simulink model "RoboBoat_SLAM_6_29"  (R2014a)
settings: Solver=FixedStepDiscrete  StartTime=0.0  StopTime=inf  FixedStep=.1  RelTol=1e-3
undefined symbols (not defined in the file): Com1, Com2, Com3, Com4, DiscIntNeverNeededParam, standard
libraries: xpcseriallib x29, visiontextngfix x25, simulink x21, slrtlib x7, speedgoatlib_IO102 x5, speedgoatlib x1
(part 5 of 6)

== matlab function RoboBoat_SLAM_6_29/Main FSM/Obstacle Navigation1/Task Option1/Message Composer ==
  data: taskStrInit input; taskStrAdj output
function taskStrAdj = composeMessage(taskStrInit)
%Written by Anderson Lebbad on August 9, 2013
%Last Edited: Edward Zhu on June 2, 2014

%This function adjusts the length of a vector to a set value by filling
%the remaining space with 0's. This is necessary for data store objects
%that have a fixed size for the memory allocation, but a variable length
%input.

%Length of message packet
strLength = 8;

%Size of text in message
taskStrLength = size(taskStrInit,1);

%Pad end of text with zeros
taskStrAdj = [taskStrInit' zeros(1,strLength-taskStrLength)];

== matlab function RoboBoat_SLAM_6_29/Main FSM/Obstacle Navigation1/GPS: Center/Orient/Within Range ==
  data: DesiredHeading input; Finished output; Compass input
function Finished = OrientLocked(DesiredHeading, Compass)

%Written by Anderson Lebbad on July 22, 2013
%Last Edited:

%This function checks to see if the target heading has been reached and 
%sends a finished signal when it has.

HeadingDiff = DesiredHeading - Compass;

%Sets the range for the difference angle to be -180 to +180
if HeadingDiff > 180
    HeadingDiff = HeadingDiff - 360;
elseif HeadingDiff < -180
    HeadingDiff = HeadingDiff + 360;
end

%If the Heading is within 3 degrees, the angle is close enough to send a
%finished signal
if abs(HeadingDiff) < 3
    Finished = 1;
else
    Finished = 0;
end

== matlab function RoboBoat_SLAM_6_29/Main FSM/Obstacle Navigation1/Obstacle Navigation/Dodge/Nav Logic ==
  data: CurrentHeading input; Dist input; Ang input; ObstDist output; RPM output; DesiredHeading output; Timer input; Timeout input; DodgeIncomplete output
 function [ObstDist, RPM, DesiredHeading, DodgeIncomplete] = NavLogic(CurrentHeading,...
    Dist, Ang, Timer, Timeout)

%Written by Anderson Lebbad on August 20, 2013
%Last Edited by:

%Determines the signals for driving through the buoy channel based on the
%bounding box and centroid signals from both the red and green detection
%blocks.

persistent TimeLastFound heldHeading

ObstDist = Dist / 100;

if isempty(TimeLastFound) && isempty(heldHeading)
    TimeLastFound = 0;
    heldHeading = CurrentHeading;
end

if ObstDist > 0 && ObstDist <= 2
    %Buffer for single buoy offset is the angle to twice the boat's width off of the
    %center of the buoy
    BoatWidth = .75;
    Buffer = atan(2 * BoatWidth / ObstDist) * 180 / pi;
    
    if Ang < 0
        ObstOffset = Ang + Buffer;
    else
        ObstOffset = Ang - Buffer;
    end
    
    DesiredHeading = mod(CurrentHeading + ObstOffset, 360);
    RPM = 2800;
    
    TimeLastFound = Timer;
    heldHeading = CurrentHeading;
    
    DodgeIncomplete = 1;
    
else
    DesiredHeading = heldHeading;
    RPM = 2800;
    
    if Timer-TimeLastFound < Timeout
        DodgeIncomplete = 1;
    else
        DodgeIncomplete = 0;
    end

end

== matlab function RoboBoat_SLAM_6_29/Sensors/1020 Comms/Data Update2 ==
  data: Valid input; ControlMode input; V output; C output; L output; A output; Data input; D1 output; D2 output; D3 output; D4 output; D5 output; D6 output; D7 output; D8 output; D9 output; D10 output; D11 output; D12 output; D13 output; D14 output; D15 output; D16 output; D17 output; D18 output; D19 output; D20 output; D21 output; D22 output; D23 output; D24 output; Activate input
function [V,C,L,A,D1,D2,D3,D4,D5,D6,D7,D8,D9,D10,D11,D12,D13,D14,D15,D16,D17,...
    D18,D19,D20,D21,D22,D23,D24] = dataSplit(Valid,ControlMode,Data,Activate)
%Written by Anderson Lebbad on August 10, 2014
%Last Edited by: Anderson Lebbad on September 11, 2014

%This function splits the data vector into the twelve channels it is
%composed of for communication

persistent HoldData

if isempty(HoldData)
    HoldData = zeros(26,1);
    HoldData(2) = 2;
end

if Valid == 1
    HoldData(1) = Valid;
    HoldData(2) = ControlMode;
    HoldData(3) = Data(1);
    HoldData(4) = Data(2);
    HoldData(5) = Data(3);
    HoldData(6) = Data(4);
    HoldData(7) = Data(5);
    HoldData(8) = Data(6);
    HoldData(9) = Data(7);
    HoldData(10) = Data(8);
    HoldData(11) = Data(9);
    HoldData(12) = Data(10);
    HoldData(13) = Data(11);
    HoldData(14) = Data(12);
    HoldData(15) = Data(13);
    HoldData(16) = Data(14);
    HoldData(17) = Data(15);
    HoldData(18) = Data(16);
    HoldData(19) = Data(17);
    HoldData(20) = Data(18);
    HoldData(21) = Data(19);
    HoldData(22) = Data(20);
    HoldData(23) = Data(21);
    HoldData(24) = Data(22);
    HoldData(25) = Data(23);
    HoldData(26) = Data(24);
end

V = HoldData(1);
C = HoldData(2);
L = 8;
A = Activate;
D1 = HoldData(3);
D2 = HoldData(4);
D3 = HoldData(5);
D4 = HoldData(6);
D5 = HoldData(7);
D6 = HoldData(8);
D7 = HoldData(9);
D8 = HoldData(10);
D9 = HoldData(11);
D10 = HoldData(12);
D11 = HoldData(13);
D12 = HoldData(14);
D13 = HoldData(15);
D14 = HoldData(16);
D15 = HoldData(17);
D16 = HoldData(18);
D17 = HoldData(19);
D18 = HoldData(20);
D19 = HoldData(21);
D20 = HoldData(22);
D21 = HoldData(23);
D22 = HoldData(24);
D23 = HoldData(25);
D24 = HoldData(26);

end

== matlab function RoboBoat_SLAM_6_29/Main FSM/Obstacle Navigation2/MATLAB Function ==
  data: requestNumOut output; CP input; requestNumIn input; Finished output
function [requestNumOut, Finished] = requestSender(CP, requestNumIn)

persistent counter
if isempty(counter)
    counter = 0;
end

if CP < 1
    requestNumOut = requestNumIn;
    Finished = 0;
else
    counter = counter + 1;
    if counter >= 50
        requestNumOut = 0;
        Finished = 1;
    else
        requestNumOut = requestNumIn;
        Finished = 0;
    end
end

== matlab function RoboBoat_SLAM_6_29/Main FSM/Shotgun Speedgate/MATLAB Function ==
  data: Heading input; LockedHeading output
function LockedHeading = HeadingLock(Heading)

persistent lock

if isempty(lock)
    lock = Heading;
end

LockedHeading = lock;

== matlab function RoboBoat_SLAM_6_29/Main FSM/Shotgun Speedgate/MATLAB Function1 ==
  data: desiredHeading input; out output; Heading input
function out = dataOrganizer(desiredHeading, Heading)
%#codegen

out = [desiredHeading Heading];

== matlab function RoboBoat_SLAM_6_29/Main FSM/SLAM/Any State Change ==
  data: u input; y output
function y = fcn(u)
%#codegen

y = any(any(u));

end

== matlab function RoboBoat_SLAM_6_29/Main FSM/SLAM/Any Landmark Change ==
  data: u input; y output
function y = fcn(u)
%#codegen

y = any(any(u));

end

== matlab function RoboBoat_SLAM_6_29/Main FSM/SLAM/SLAM enabled/Part Pos ==
  data: particle_pose output; part_positions input
function particle_pose   = partPos( part_positions )
%Written by Anderson Lebbad on March 16, 2015
%Last Edited:
%
%This function reorganizes the particle positions row wise by particle,
%columns being X,Y,Psi

particle_pose = nan(50,3);

particle_pose(:,1) = part_positions(1:3:150);
particle_pose(:,2) = part_positions(2:3:150);
particle_pose(:,3) = part_positions(3:3:150);

end

== matlab function RoboBoat_SLAM_6_29/Main FSM/SLAM/SLAM enabled/dataMat ==
  data: lm_data_mat output; lm_data input
function lm_data_mat   = dataMat( lm_data )
%Written by Anderson Lebbad on March 16, 2015
%Last Edited:
%
%This function reorganizes the particle positions row wise by particle,
%columns being X,Y,Psi

lm_data_mat = nan(12,2);

lm_data_mat(:,1) = lm_data(1:2:24);
lm_data_mat(:,2) = lm_data(2:2:24);

end

== matlab function RoboBoat_SLAM_6_29/Main FSM/SLAM/inputselection/MATLAB Function ==
  data: Landmarkchange input; controlchange input; xypsi input; part_positions input; x50 output; xypsi150 input; y50 output; psi50 output
function [x50, y50, psi50] = fcn(Landmarkchange,controlchange,xypsi,part_positions,xypsi150)

%Preallocate output
x50 = zeros(50,1);
y50 = zeros(50,1);
psi50 = zeros(50,1);
%Check to see how output shoud be assigned
if (Landmarkchange==1)
    x50 = part_positions(1:3:150);
    y50 = part_positions(2:3:150);
    psi50 = part_positions(3:3:150);
elseif (controlchange==1)
    %Assign current state to all
    x50(:) = xypsi(1);
    y50(:) = xypsi(2);
    psi50(:) = xypsi(3);
else
    x50 = xypsi150(1:3:150);
    y50 = xypsi150(2:3:150);
    psi50 = xypsi150(3:3:150);
end

end

== system RoboBoat_SLAM_6_29/Main FSM/SLAM/Models for prediction/Model37 ==
  X : Inport
  Y : Inport  Port=2
  Psi : Inport  Port=3
  Nav Messages : Inport  Port=4
  Bus Creator : BusCreator  Inputs=3
  Bus Selector : BusSelector  OutputSignals=IMU.Velocity.u,IMU.Velocity.v,IMU.Rate of Turn.GyrZ,Thrust.PortPow,Thrust.StbdPow
  Model : ModelReference  ModelNameDialog=SeaCat_Dynamic_Model.slx  SimulationMode=Normal  ModelReferenceVersion=1.2137  CopyOfModelName=SeaCat_Dynamic_Model.slx  DefaultDataLogging=on
  No Azimuth : Constant  Value=0
  NEyaw : Outport
  wires:
  Nav Messages/1 -> Bus Selector/1
  X/1 -> Model/1
  Y/1 -> Model/2
  Psi/1 -> Model/3
  Bus Selector/1 -> Model/4  "<u>"
  Bus Selector/2 -> Model/5  "<v>"
  Bus Selector/3 -> Model/6  "<GyrZ>"
  Bus Selector/4 -> Model/7  "<PortPow>"
  Bus Selector/5 -> Model/9  "<StbdPow>"
  No Azimuth/1 -> Model/8, Model/10
  Model/1 -> Bus Creator/1  "N"
  Model/3 -> Bus Creator/3  "yaw"
  Model/2 -> Bus Creator/2  "E"
  Bus Creator/1 -> NEyaw/1

== system RoboBoat_SLAM_6_29/Main FSM/SLAM/Models for prediction/Model38 ==
  X : Inport
  Y : Inport  Port=2
  Psi : Inport  Port=3
  Nav Messages : Inport  Port=4
  Bus Creator : BusCreator  Inputs=3
  Bus Selector : BusSelector  OutputSignals=IMU.Velocity.u,IMU.Velocity.v,IMU.Rate of Turn.GyrZ,Thrust.PortPow,Thrust.StbdPow
  Model : ModelReference  ModelNameDialog=SeaCat_Dynamic_Model.slx  SimulationMode=Normal  ModelReferenceVersion=1.2137  CopyOfModelName=SeaCat_Dynamic_Model.slx  DefaultDataLogging=on
  No Azimuth : Constant  Value=0
  NEyaw : Outport
  wires:
  Nav Messages/1 -> Bus Selector/1
  X/1 -> Model/1
  Y/1 -> Model/2
  Psi/1 -> Model/3
  Bus Selector/1 -> Model/4  "<u>"
  Bus Selector/2 -> Model/5  "<v>"
  Bus Selector/3 -> Model/6  "<GyrZ>"
  Bus Selector/4 -> Model/7  "<PortPow>"
  Bus Selector/5 -> Model/9  "<StbdPow>"
  No Azimuth/1 -> Model/8, Model/10
  Model/1 -> Bus Creator/1  "N"
  Model/3 -> Bus Creator/3  "yaw"
  Model/2 -> Bus Creator/2  "E"
  Bus Creator/1 -> NEyaw/1

== system RoboBoat_SLAM_6_29/Main FSM/SLAM/Models for prediction/Model39 ==
  X : Inport
  Y : Inport  Port=2
  Psi : Inport  Port=3
  Nav Messages : Inport  Port=4
  Bus Creator : BusCreator  Inputs=3
  Bus Selector : BusSelector  OutputSignals=IMU.Velocity.u,IMU.Velocity.v,IMU.Rate of Turn.GyrZ,Thrust.PortPow,Thrust.StbdPow
  Model : ModelReference  ModelNameDialog=SeaCat_Dynamic_Model.slx  SimulationMode=Normal  ModelReferenceVersion=1.2137  CopyOfModelName=SeaCat_Dynamic_Model.slx  DefaultDataLogging=on
  No Azimuth : Constant  Value=0
  NEyaw : Outport
  wires:
  Nav Messages/1 -> Bus Selector/1
  X/1 -> Model/1
  Y/1 -> Model/2
  Psi/1 -> Model/3
  Bus Selector/1 -> Model/4  "<u>"
  Bus Selector/2 -> Model/5  "<v>"
  Bus Selector/3 -> Model/6  "<GyrZ>"
  Bus Selector/4 -> Model/7  "<PortPow>"
  Bus Selector/5 -> Model/9  "<StbdPow>"
  No Azimuth/1 -> Model/8, Model/10
  Model/1 -> Bus Creator/1  "N"
  Model/3 -> Bus Creator/3  "yaw"
  Model/2 -> Bus Creator/2  "E"
  Bus Creator/1 -> NEyaw/1

== system RoboBoat_SLAM_6_29/Main FSM/SLAM/Models for prediction/Model4 ==
  X : Inport
  Y : Inport  Port=2
  Psi : Inport  Port=3
  Nav Messages : Inport  Port=4
  Bus Creator : BusCreator  Inputs=3
  Bus Selector : BusSelector  OutputSignals=IMU.Velocity.u,IMU.Velocity.v,IMU.Rate of Turn.GyrZ,Thrust.PortPow,Thrust.StbdPow
  Model : ModelReference  ModelNameDialog=SeaCat_Dynamic_Model.slx  SimulationMode=Normal  ModelReferenceVersion=1.2137  CopyOfModelName=SeaCat_Dynamic_Model.slx  DefaultDataLogging=on
  No Azimuth : Constant  Value=0
  NEyaw : Outport
  wires:
  Nav Messages/1 -> Bus Selector/1
  X/1 -> Model/1
  Y/1 -> Model/2
  Psi/1 -> Model/3
  Bus Selector/1 -> Model/4  "<u>"
  Bus Selector/2 -> Model/5  "<v>"
  Bus Selector/3 -> Model/6  "<GyrZ>"
  Bus Selector/4 -> Model/7  "<PortPow>"
  Bus Selector/5 -> Model/9  "<StbdPow>"
  No Azimuth/1 -> Model/8, Model/10
  Model/1 -> Bus Creator/1  "N"
  Model/3 -> Bus Creator/3  "yaw"
  Model/2 -> Bus Creator/2  "E"
  Bus Creator/1 -> NEyaw/1

== system RoboBoat_SLAM_6_29/Main FSM/SLAM/Models for prediction/Model40 ==
  X : Inport
  Y : Inport  Port=2
  Psi : Inport  Port=3
  Nav Messages : Inport  Port=4
  Bus Creator : BusCreator  Inputs=3
  Bus Selector : BusSelector  OutputSignals=IMU.Velocity.u,IMU.Velocity.v,IMU.Rate of Turn.GyrZ,Thrust.PortPow,Thrust.StbdPow
  Model : ModelReference  ModelNameDialog=SeaCat_Dynamic_Model.slx  SimulationMode=Normal  ModelReferenceVersion=1.2137  CopyOfModelName=SeaCat_Dynamic_Model.slx  DefaultDataLogging=on
  No Azimuth : Constant  Value=0
  NEyaw : Outport
  wires:
  Nav Messages/1 -> Bus Selector/1
  X/1 -> Model/1
  Y/1 -> Model/2
  Psi/1 -> Model/3
  Bus Selector/1 -> Model/4  "<u>"
  Bus Selector/2 -> Model/5  "<v>"
  Bus Selector/3 -> Model/6  "<GyrZ>"
  Bus Selector/4 -> Model/7  "<PortPow>"
  Bus Selector/5 -> Model/9  "<StbdPow>"
  No Azimuth/1 -> Model/8, Model/10
  Model/1 -> Bus Creator/1  "N"
  Model/3 -> Bus Creator/3  "yaw"
  Model/2 -> Bus Creator/2  "E"
  Bus Creator/1 -> NEyaw/1

== system RoboBoat_SLAM_6_29/Main FSM/SLAM/Models for prediction/Model41 ==
  X : Inport
  Y : Inport  Port=2
  Psi : Inport  Port=3
  Nav Messages : Inport  Port=4
  Bus Creator : BusCreator  Inputs=3
  Bus Selector : BusSelector  OutputSignals=IMU.Velocity.u,IMU.Velocity.v,IMU.Rate of Turn.GyrZ,Thrust.PortPow,Thrust.StbdPow
  Model : ModelReference  ModelNameDialog=SeaCat_Dynamic_Model.slx  SimulationMode=Normal  ModelReferenceVersion=1.2137  CopyOfModelName=SeaCat_Dynamic_Model.slx  DefaultDataLogging=on
  No Azimuth : Constant  Value=0
  NEyaw : Outport
  wires:
  Nav Messages/1 -> Bus Selector/1
  X/1 -> Model/1
  Y/1 -> Model/2
  Psi/1 -> Model/3
  Bus Selector/1 -> Model/4  "<u>"
  Bus Selector/2 -> Model/5  "<v>"
  Bus Selector/3 -> Model/6  "<GyrZ>"
  Bus Selector/4 -> Model/7  "<PortPow>"
  Bus Selector/5 -> Model/9  "<StbdPow>"
  No Azimuth/1 -> Model/8, Model/10
  Model/1 -> Bus Creator/1  "N"
  Model/3 -> Bus Creator/3  "yaw"
  Model/2 -> Bus Creator/2  "E"
  Bus Creator/1 -> NEyaw/1

== system RoboBoat_SLAM_6_29/Main FSM/SLAM/Models for prediction/Model42 ==
  X : Inport
  Y : Inport  Port=2
  Psi : Inport  Port=3
  Nav Messages : Inport  Port=4
  Bus Creator : BusCreator  Inputs=3
  Bus Selector : BusSelector  OutputSignals=IMU.Velocity.u,IMU.Velocity.v,IMU.Rate of Turn.GyrZ,Thrust.PortPow,Thrust.StbdPow
  Model : ModelReference  ModelNameDialog=SeaCat_Dynamic_Model.slx  SimulationMode=Normal  ModelReferenceVersion=1.2137  CopyOfModelName=SeaCat_Dynamic_Model.slx  DefaultDataLogging=on
  No Azimuth : Constant  Value=0
  NEyaw : Outport
  wires:
  Nav Messages/1 -> Bus Selector/1
  X/1 -> Model/1
  Y/1 -> Model/2
  Psi/1 -> Model/3
  Bus Selector/1 -> Model/4  "<u>"
  Bus Selector/2 -> Model/5  "<v>"
  Bus Selector/3 -> Model/6  "<GyrZ>"
  Bus Selector/4 -> Model/7  "<PortPow>"
  Bus Selector/5 -> Model/9  "<StbdPow>"
  No Azimuth/1 -> Model/8, Model/10
  Model/1 -> Bus Creator/1  "N"
  Model/3 -> Bus Creator/3  "yaw"
  Model/2 -> Bus Creator/2  "E"
  Bus Creator/1 -> NEyaw/1

== system RoboBoat_SLAM_6_29/Main FSM/SLAM/Models for prediction/Model43 ==
  X : Inport
  Y : Inport  Port=2
  Psi : Inport  Port=3
  Nav Messages : Inport  Port=4
  Bus Creator : BusCreator  Inputs=3
  Bus Selector : BusSelector  OutputSignals=IMU.Velocity.u,IMU.Velocity.v,IMU.Rate of Turn.GyrZ,Thrust.PortPow,Thrust.StbdPow
  Model : ModelReference  ModelNameDialog=SeaCat_Dynamic_Model.slx  SimulationMode=Normal  ModelReferenceVersion=1.2137  CopyOfModelName=SeaCat_Dynamic_Model.slx  DefaultDataLogging=on
  No Azimuth : Constant  Value=0
  NEyaw : Outport
  wires:
  Nav Messages/1 -> Bus Selector/1
  X/1 -> Model/1
  Y/1 -> Model/2
  Psi/1 -> Model/3
  Bus Selector/1 -> Model/4  "<u>"
  Bus Selector/2 -> Model/5  "<v>"
  Bus Selector/3 -> Model/6  "<GyrZ>"
  Bus Selector/4 -> Model/7  "<PortPow>"
  Bus Selector/5 -> Model/9  "<StbdPow>"
  No Azimuth/1 -> Model/8, Model/10
  Model/1 -> Bus Creator/1  "N"
  Model/3 -> Bus Creator/3  "yaw"
  Model/2 -> Bus Creator/2  "E"
  Bus Creator/1 -> NEyaw/1

== system RoboBoat_SLAM_6_29/Main FSM/SLAM/Models for prediction/Model44 ==
  X : Inport
  Y : Inport  Port=2
  Psi : Inport  Port=3
  Nav Messages : Inport  Port=4
  Bus Creator : BusCreator  Inputs=3
  Bus Selector : BusSelector  OutputSignals=IMU.Velocity.u,IMU.Velocity.v,IMU.Rate of Turn.GyrZ,Thrust.PortPow,Thrust.StbdPow
  Model : ModelReference  ModelNameDialog=SeaCat_Dynamic_Model.slx  SimulationMode=Normal  ModelReferenceVersion=1.2137  CopyOfModelName=SeaCat_Dynamic_Model.slx  DefaultDataLogging=on
  No Azimuth : Constant  Value=0
  NEyaw : Outport
  wires:
  Nav Messages/1 -> Bus Selector/1
  X/1 -> Model/1
  Y/1 -> Model/2
  Psi/1 -> Model/3
  Bus Selector/1 -> Model/4  "<u>"
  Bus Selector/2 -> Model/5  "<v>"
  Bus Selector/3 -> Model/6  "<GyrZ>"
  Bus Selector/4 -> Model/7  "<PortPow>"
  Bus Selector/5 -> Model/9  "<StbdPow>"
  No Azimuth/1 -> Model/8, Model/10
  Model/1 -> Bus Creator/1  "N"
  Model/3 -> Bus Creator/3  "yaw"
  Model/2 -> Bus Creator/2  "E"
  Bus Creator/1 -> NEyaw/1

== system RoboBoat_SLAM_6_29/Main FSM/SLAM/Models for prediction/Model45 ==
  X : Inport
  Y : Inport  Port=2
  Psi : Inport  Port=3
  Nav Messages : Inport  Port=4
  Bus Creator : BusCreator  Inputs=3
  Bus Selector : BusSelector  OutputSignals=IMU.Velocity.u,IMU.Velocity.v,IMU.Rate of Turn.GyrZ,Thrust.PortPow,Thrust.StbdPow
  Model : ModelReference  ModelNameDialog=SeaCat_Dynamic_Model.slx  SimulationMode=Normal  ModelReferenceVersion=1.2137  CopyOfModelName=SeaCat_Dynamic_Model.slx  DefaultDataLogging=on
  No Azimuth : Constant  Value=0
  NEyaw : Outport
  wires:
  Nav Messages/1 -> Bus Selector/1
  X/1 -> Model/1
  Y/1 -> Model/2
  Psi/1 -> Model/3
  Bus Selector/1 -> Model/4  "<u>"
  Bus Selector/2 -> Model/5  "<v>"
  Bus Selector/3 -> Model/6  "<GyrZ>"
  Bus Selector/4 -> Model/7  "<PortPow>"
  Bus Selector/5 -> Model/9  "<StbdPow>"
  No Azimuth/1 -> Model/8, Model/10
  Model/1 -> Bus Creator/1  "N"
  Model/3 -> Bus Creator/3  "yaw"
  Model/2 -> Bus Creator/2  "E"
  Bus Creator/1 -> NEyaw/1

== system RoboBoat_SLAM_6_29/Main FSM/SLAM/Models for prediction/Model46 ==
  X : Inport
  Y : Inport  Port=2
  Psi : Inport  Port=3
  Nav Messages : Inport  Port=4
  Bus Creator : BusCreator  Inputs=3
  Bus Selector : BusSelector  OutputSignals=IMU.Velocity.u,IMU.Velocity.v,IMU.Rate of Turn.GyrZ,Thrust.PortPow,Thrust.StbdPow
  Model : ModelReference  ModelNameDialog=SeaCat_Dynamic_Model.slx  SimulationMode=Normal  ModelReferenceVersion=1.2137  CopyOfModelName=SeaCat_Dynamic_Model.slx  DefaultDataLogging=on
  No Azimuth : Constant  Value=0
  NEyaw : Outport
  wires:
  Nav Messages/1 -> Bus Selector/1
  X/1 -> Model/1
  Y/1 -> Model/2
  Psi/1 -> Model/3
  Bus Selector/1 -> Model/4  "<u>"
  Bus Selector/2 -> Model/5  "<v>"
  Bus Selector/3 -> Model/6  "<GyrZ>"
  Bus Selector/4 -> Model/7  "<PortPow>"
  Bus Selector/5 -> Model/9  "<StbdPow>"
  No Azimuth/1 -> Model/8, Model/10
  Model/1 -> Bus Creator/1  "N"
  Model/3 -> Bus Creator/3  "yaw"
  Model/2 -> Bus Creator/2  "E"
  Bus Creator/1 -> NEyaw/1

== system RoboBoat_SLAM_6_29/Main FSM/SLAM/Models for prediction/Model47 ==
  X : Inport
  Y : Inport  Port=2
  Psi : Inport  Port=3
  Nav Messages : Inport  Port=4
  Bus Creator : BusCreator  Inputs=3
  Bus Selector : BusSelector  OutputSignals=IMU.Velocity.u,IMU.Velocity.v,IMU.Rate of Turn.GyrZ,Thrust.PortPow,Thrust.StbdPow
  Model : ModelReference  ModelNameDialog=SeaCat_Dynamic_Model.slx  SimulationMode=Normal  ModelReferenceVersion=1.2137  CopyOfModelName=SeaCat_Dynamic_Model.slx  DefaultDataLogging=on
  No Azimuth : Constant  Value=0
  NEyaw : Outport
  wires:
  Nav Messages/1 -> Bus Selector/1
  X/1 -> Model/1
  Y/1 -> Model/2
  Psi/1 -> Model/3
  Bus Selector/1 -> Model/4  "<u>"
  Bus Selector/2 -> Model/5  "<v>"
  Bus Selector/3 -> Model/6  "<GyrZ>"
  Bus Selector/4 -> Model/7  "<PortPow>"
  Bus Selector/5 -> Model/9  "<StbdPow>"
  No Azimuth/1 -> Model/8, Model/10
  Model/1 -> Bus Creator/1  "N"
  Model/3 -> Bus Creator/3  "yaw"
  Model/2 -> Bus Creator/2  "E"
  Bus Creator/1 -> NEyaw/1

== system RoboBoat_SLAM_6_29/Main FSM/SLAM/Models for prediction/Model48 ==
  X : Inport
  Y : Inport  Port=2
  Psi : Inport  Port=3
  Nav Messages : Inport  Port=4
  Bus Creator : BusCreator  Inputs=3
  Bus Selector : BusSelector  OutputSignals=IMU.Velocity.u,IMU.Velocity.v,IMU.Rate of Turn.GyrZ,Thrust.PortPow,Thrust.StbdPow
  Model : ModelReference  ModelNameDialog=SeaCat_Dynamic_Model.slx  SimulationMode=Normal  ModelReferenceVersion=1.2137  CopyOfModelName=SeaCat_Dynamic_Model.slx  DefaultDataLogging=on
  No Azimuth : Constant  Value=0
  NEyaw : Outport
  wires:
  Nav Messages/1 -> Bus Selector/1
  X/1 -> Model/1
  Y/1 -> Model/2
  Psi/1 -> Model/3
  Bus Selector/1 -> Model/4  "<u>"
  Bus Selector/2 -> Model/5  "<v>"
  Bus Selector/3 -> Model/6  "<GyrZ>"
  Bus Selector/4 -> Model/7  "<PortPow>"
  Bus Selector/5 -> Model/9  "<StbdPow>"
  No Azimuth/1 -> Model/8, Model/10
  Model/1 -> Bus Creator/1  "N"
  Model/3 -> Bus Creator/3  "yaw"
  Model/2 -> Bus Creator/2  "E"
  Bus Creator/1 -> NEyaw/1

== system RoboBoat_SLAM_6_29/Main FSM/SLAM/Models for prediction/Model49 ==
  X : Inport
  Y : Inport  Port=2
  Psi : Inport  Port=3
  Nav Messages : Inport  Port=4
  Bus Creator : BusCreator  Inputs=3
  Bus Selector : BusSelector  OutputSignals=IMU.Velocity.u,IMU.Velocity.v,IMU.Rate of Turn.GyrZ,Thrust.PortPow,Thrust.StbdPow
  Model : ModelReference  ModelNameDialog=SeaCat_Dynamic_Model.slx  SimulationMode=Normal  ModelReferenceVersion=1.2137  CopyOfModelName=SeaCat_Dynamic_Model.slx  DefaultDataLogging=on
  No Azimuth : Constant  Value=0
  NEyaw : Outport
  wires:
  Nav Messages/1 -> Bus Selector/1
  X/1 -> Model/1
  Y/1 -> Model/2
  Psi/1 -> Model/3
  Bus Selector/1 -> Model/4  "<u>"
  Bus Selector/2 -> Model/5  "<v>"
  Bus Selector/3 -> Model/6  "<GyrZ>"
  Bus Selector/4 -> Model/7  "<PortPow>"
  Bus Selector/5 -> Model/9  "<StbdPow>"
  No Azimuth/1 -> Model/8, Model/10
  Model/1 -> Bus Creator/1  "N"
  Model/3 -> Bus Creator/3  "yaw"
  Model/2 -> Bus Creator/2  "E"
  Bus Creator/1 -> NEyaw/1

== system RoboBoat_SLAM_6_29/Main FSM/SLAM/Models for prediction/Model5 ==
  X : Inport
  Y : Inport  Port=2
  Psi : Inport  Port=3
  Nav Messages : Inport  Port=4
  Bus Creator : BusCreator  Inputs=3
  Bus Selector : BusSelector  OutputSignals=IMU.Velocity.u,IMU.Velocity.v,IMU.Rate of Turn.GyrZ,Thrust.PortPow,Thrust.StbdPow
  Model : ModelReference  ModelNameDialog=SeaCat_Dynamic_Model.slx  SimulationMode=Normal  ModelReferenceVersion=1.2137  CopyOfModelName=SeaCat_Dynamic_Model.slx  DefaultDataLogging=on
  No Azimuth : Constant  Value=0
  NEyaw : Outport
  wires:
  Nav Messages/1 -> Bus Selector/1
  X/1 -> Model/1
  Y/1 -> Model/2
  Psi/1 -> Model/3
  Bus Selector/1 -> Model/4  "<u>"
  Bus Selector/2 -> Model/5  "<v>"
  Bus Selector/3 -> Model/6  "<GyrZ>"
  Bus Selector/4 -> Model/7  "<PortPow>"
  Bus Selector/5 -> Model/9  "<StbdPow>"
  No Azimuth/1 -> Model/8, Model/10
  Model/1 -> Bus Creator/1  "N"
  Model/3 -> Bus Creator/3  "yaw"
  Model/2 -> Bus Creator/2  "E"
  Bus Creator/1 -> NEyaw/1

== system RoboBoat_SLAM_6_29/Main FSM/SLAM/Models for prediction/Model50 ==
  X : Inport
  Y : Inport  Port=2
  Psi : Inport  Port=3
  Nav Messages : Inport  Port=4
  Bus Creator : BusCreator  Inputs=3
  Bus Selector : BusSelector  OutputSignals=IMU.Velocity.u,IMU.Velocity.v,IMU.Rate of Turn.GyrZ,Thrust.PortPow,Thrust.StbdPow
  Model : ModelReference  ModelNameDialog=SeaCat_Dynamic_Model.slx  SimulationMode=Normal  ModelReferenceVersion=1.2137  CopyOfModelName=SeaCat_Dynamic_Model.slx  DefaultDataLogging=on
  No Azimuth : Constant  Value=0
  NEyaw : Outport
  wires:
  Nav Messages/1 -> Bus Selector/1
  X/1 -> Model/1
  Y/1 -> Model/2
  Psi/1 -> Model/3
  Bus Selector/1 -> Model/4  "<u>"
  Bus Selector/2 -> Model/5  "<v>"
  Bus Selector/3 -> Model/6  "<GyrZ>"
  Bus Selector/4 -> Model/7  "<PortPow>"
  Bus Selector/5 -> Model/9  "<StbdPow>"
  No Azimuth/1 -> Model/8, Model/10
  Model/1 -> Bus Creator/1  "N"
  Model/3 -> Bus Creator/3  "yaw"
  Model/2 -> Bus Creator/2  "E"
  Bus Creator/1 -> NEyaw/1

== system RoboBoat_SLAM_6_29/Main FSM/SLAM/Models for prediction/Model6 ==
  X : Inport
  Y : Inport  Port=2
  Psi : Inport  Port=3
  Nav Messages : Inport  Port=4
  Bus Creator : BusCreator  Inputs=3
  Bus Selector : BusSelector  OutputSignals=IMU.Velocity.u,IMU.Velocity.v,IMU.Rate of Turn.GyrZ,Thrust.PortPow,Thrust.StbdPow
  Model : ModelReference  ModelNameDialog=SeaCat_Dynamic_Model.slx  SimulationMode=Normal  ModelReferenceVersion=1.2137  CopyOfModelName=SeaCat_Dynamic_Model.slx  DefaultDataLogging=on
  No Azimuth : Constant  Value=0
  NEyaw : Outport
  wires:
  Nav Messages/1 -> Bus Selector/1
  X/1 -> Model/1
  Y/1 -> Model/2
  Psi/1 -> Model/3
  Bus Selector/1 -> Model/4  "<u>"
  Bus Selector/2 -> Model/5  "<v>"
  Bus Selector/3 -> Model/6  "<GyrZ>"
  Bus Selector/4 -> Model/7  "<PortPow>"
  Bus Selector/5 -> Model/9  "<StbdPow>"
  No Azimuth/1 -> Model/8, Model/10
  Model/1 -> Bus Creator/1  "N"
  Model/3 -> Bus Creator/3  "yaw"
  Model/2 -> Bus Creator/2  "E"
  Bus Creator/1 -> NEyaw/1

== system RoboBoat_SLAM_6_29/Main FSM/SLAM/Models for prediction/Model7 ==
  X : Inport
  Y : Inport  Port=2
  Psi : Inport  Port=3
  Nav Messages : Inport  Port=4
  Bus Creator : BusCreator  Inputs=3
  Bus Selector : BusSelector  OutputSignals=IMU.Velocity.u,IMU.Velocity.v,IMU.Rate of Turn.GyrZ,Thrust.PortPow,Thrust.StbdPow
  Model : ModelReference  ModelNameDialog=SeaCat_Dynamic_Model.slx  SimulationMode=Normal  ModelReferenceVersion=1.2137  CopyOfModelName=SeaCat_Dynamic_Model.slx  DefaultDataLogging=on
  No Azimuth : Constant  Value=0
  NEyaw : Outport
  wires:
  Nav Messages/1 -> Bus Selector/1
  X/1 -> Model/1
  Y/1 -> Model/2
  Psi/1 -> Model/3
  Bus Selector/1 -> Model/4  "<u>"
  Bus Selector/2 -> Model/5  "<v>"
  Bus Selector/3 -> Model/6  "<GyrZ>"
  Bus Selector/4 -> Model/7  "<PortPow>"
  Bus Selector/5 -> Model/9  "<StbdPow>"
  No Azimuth/1 -> Model/8, Model/10
  Model/1 -> Bus Creator/1  "N"
  Model/3 -> Bus Creator/3  "yaw"
  Model/2 -> Bus Creator/2  "E"
  Bus Creator/1 -> NEyaw/1

== system RoboBoat_SLAM_6_29/Main FSM/SLAM/Models for prediction/Model8 ==
  X : Inport
  Y : Inport  Port=2
  Psi : Inport  Port=3
  Nav Messages : Inport  Port=4
  Bus Creator : BusCreator  Inputs=3
  Bus Selector : BusSelector  OutputSignals=IMU.Velocity.u,IMU.Velocity.v,IMU.Rate of Turn.GyrZ,Thrust.PortPow,Thrust.StbdPow
  Model : ModelReference  ModelNameDialog=SeaCat_Dynamic_Model.slx  SimulationMode=Normal  ModelReferenceVersion=1.2137  CopyOfModelName=SeaCat_Dynamic_Model.slx  DefaultDataLogging=on
  No Azimuth : Constant  Value=0
  NEyaw : Outport
  wires:
  Nav Messages/1 -> Bus Selector/1
  X/1 -> Model/1
  Y/1 -> Model/2
  Psi/1 -> Model/3
  Bus Selector/1 -> Model/4  "<u>"
  Bus Selector/2 -> Model/5  "<v>"
  Bus Selector/3 -> Model/6  "<GyrZ>"
  Bus Selector/4 -> Model/7  "<PortPow>"
  Bus Selector/5 -> Model/9  "<StbdPow>"
  No Azimuth/1 -> Model/8, Model/10
  Model/1 -> Bus Creator/1  "N"
  Model/3 -> Bus Creator/3  "yaw"
  Model/2 -> Bus Creator/2  "E"
  Bus Creator/1 -> NEyaw/1

== system RoboBoat_SLAM_6_29/Main FSM/SLAM/Models for prediction/Model9 ==
  X : Inport
  Y : Inport  Port=2
  Psi : Inport  Port=3
  Nav Messages : Inport  Port=4
  Bus Creator : BusCreator  Inputs=3
  Bus Selector : BusSelector  OutputSignals=IMU.Velocity.u,IMU.Velocity.v,IMU.Rate of Turn.GyrZ,Thrust.PortPow,Thrust.StbdPow
  Model : ModelReference  ModelNameDialog=SeaCat_Dynamic_Model.slx  SimulationMode=Normal  ModelReferenceVersion=1.2137  CopyOfModelName=SeaCat_Dynamic_Model.slx  DefaultDataLogging=on
  No Azimuth : Constant  Value=0
  NEyaw : Outport
  wires:
  Nav Messages/1 -> Bus Selector/1
  X/1 -> Model/1
  Y/1 -> Model/2
  Psi/1 -> Model/3
  Bus Selector/1 -> Model/4  "<u>"
  Bus Selector/2 -> Model/5  "<v>"
  Bus Selector/3 -> Model/6  "<GyrZ>"
  Bus Selector/4 -> Model/7  "<PortPow>"
  Bus Selector/5 -> Model/9  "<StbdPow>"
  No Azimuth/1 -> Model/8, Model/10
  Model/1 -> Bus Creator/1  "N"
  Model/3 -> Bus Creator/3  "yaw"
  Model/2 -> Bus Creator/2  "E"
  Bus Creator/1 -> NEyaw/1

== system RoboBoat_SLAM_6_29/Main FSM/Start Speed/Gate Find and Through/Find ==
  Sensors : Inport
  Enable : EnablePort
  Bus Selector : BusSelector  OutputSignals=LIDAR.Landmarks.Distances,LIDAR.Landmarks.Angles,IMU.Position.X,IMU.Position.Y,IMU.Orientation.Yaw
  MATLAB Function1 : MATLAB Function  TreatAsAtomicUnit=on
  Output Heirarchy : Subsystem
  RPM : Constant  Value=0  SampleTime=-1
  Write : DataStoreWrite  DataStoreName=GateNED
  Outputs : Outport
  Finished : Outport  Port=2
  wires:
  Output Heirarchy/1(Outputs) -> Outputs/1
  RPM/1 -> Output Heirarchy/2(RPM)
  MATLAB Function1/2(Goal) -> Write/1
  MATLAB Function1/1(found) -> Finished/1
  MATLAB Function1/3(DesiredHeading) -> Output Heirarchy/3(Desired Heading)
  Sensors/1 -> Output Heirarchy/1(Sensors), Bus Selector/1  "Sensors"
  Bus Selector/1 -> MATLAB Function1/1(Dist)  "<Distances>"
  Bus Selector/3 -> MATLAB Function1/3(X)  "<X>"
  Bus Selector/2 -> MATLAB Function1/2(Angles)  "<Angles>"
  Bus Selector/4 -> MATLAB Function1/4(Y)  "<Y>"
  Bus Selector/5 -> MATLAB Function1/5(Heading)  "<Yaw>"

== system RoboBoat_SLAM_6_29/Main FSM/Start Speed/Gate Find and Through/Through ==
  Sensors : Inport
  Enable : EnablePort
  Bus Selector2 : BusSelector  OutputSignals=IMU.Position.X,IMU.Position.Y,IMU.Orientation.Yaw
  Data Store Read3 : DataStoreRead  DataStoreName=GateNED
  Demux : Demux  Outputs=2
  Model : ModelReference  ModelNameDialog=NEDnavV5.slx  SimulationMode=Normal  ModelReferenceVersion=1.2059  CopyOfModelName=NEDnavV5.slx  DefaultDataLogging=on
  Output Heirarchy : Subsystem
  Outputs : Outport
  Finished : Outport  Port=2
  wires:
  Model/1 -> Output Heirarchy/2(RPM)
  Model/2 -> Output Heirarchy/3(Desired Heading)
  Model/3 -> Finished/1
  Output Heirarchy/1(Outputs) -> Outputs/1
  Sensors/1 -> Bus Selector2/1, Output Heirarchy/1(Sensors)
  Bus Selector2/1 -> Model/1  "<X>"
  Bus Selector2/2 -> Model/2  "<Y>"
  Bus Selector2/3 -> Model/3  "<Yaw>"
  Data Store Read3/1 -> Demux/1
  Demux/1 -> Model/4
  Demux/2 -> Model/5

== system RoboBoat_SLAM_6_29/Main FSM/Start Speed/Gate Find and Through1/Find ==
  Sensors : Inport
  Enable : EnablePort
  Bus Selector : BusSelector  OutputSignals=LIDAR.Landmarks.Distances,LIDAR.Landmarks.Angles,IMU.Position.X,IMU.Position.Y,IMU.Orientation.Yaw
  MATLAB Function1 : MATLAB Function  TreatAsAtomicUnit=on
  Output Heirarchy : Subsystem
  RPM : Constant  Value=0  SampleTime=-1
  Write : DataStoreWrite  DataStoreName=GateNED
  Outputs : Outport
  Finished : Outport  Port=2
  wires:
  Output Heirarchy/1(Outputs) -> Outputs/1
  RPM/1 -> Output Heirarchy/2(RPM)
  MATLAB Function1/2(Goal) -> Write/1
  MATLAB Function1/1(found) -> Finished/1
  MATLAB Function1/3(DesiredHeading) -> Output Heirarchy/3(Desired Heading)
  Sensors/1 -> Output Heirarchy/1(Sensors), Bus Selector/1  "Sensors"
  Bus Selector/1 -> MATLAB Function1/1(Dist)  "<Distances>"
  Bus Selector/3 -> MATLAB Function1/3(X)  "<X>"
  Bus Selector/2 -> MATLAB Function1/2(Angles)  "<Angles>"
  Bus Selector/4 -> MATLAB Function1/4(Y)  "<Y>"
  Bus Selector/5 -> MATLAB Function1/5(Heading)  "<Yaw>"

== system RoboBoat_SLAM_6_29/Main FSM/Start Speed/Gate Find and Through1/Through ==
  Sensors : Inport
  Enable : EnablePort
  Bus Selector2 : BusSelector  OutputSignals=IMU.Position.X,IMU.Position.Y,IMU.Orientation.Yaw
  Data Store Read3 : DataStoreRead  DataStoreName=GateNED
  Demux : Demux  Outputs=2
  Model : ModelReference  ModelNameDialog=NEDnavV5.slx  SimulationMode=Normal  ModelReferenceVersion=1.2059  CopyOfModelName=NEDnavV5.slx  DefaultDataLogging=on
  Output Heirarchy : Subsystem
  Outputs : Outport
  Finished : Outport  Port=2
  wires:
  Model/1 -> Output Heirarchy/2(RPM)
  Model/2 -> Output Heirarchy/3(Desired Heading)
  Model/3 -> Finished/1
  Output Heirarchy/1(Outputs) -> Outputs/1
  Sensors/1 -> Bus Selector2/1, Output Heirarchy/1(Sensors)
  Bus Selector2/1 -> Model/1  "<X>"
  Bus Selector2/2 -> Model/2  "<Y>"
  Bus Selector2/3 -> Model/3  "<Yaw>"
  Data Store Read3/1 -> Demux/1
  Demux/1 -> Model/4
  Demux/2 -> Model/5

== system RoboBoat_SLAM_6_29/Main FSM/Obstacle Navigation1/Enter Gate/Gate 1 (Red & White)/Output Heirarchy ==
  Annotated Image : Inport
  Sensors : Inport  Port=2
  RPM : Inport  Port=3
  Desired Heading : Inport  Port=4
  Task Finished : Inport  Port=5
  Bus Creator : BusCreator  Inputs=3
  Bus Creator1 : BusCreator  Inputs=2
  Bus Creator2 : BusCreator  Inputs=3
  Bus Creator3 : BusCreator  Inputs=2
  Bus Creator4 : BusCreator  Inputs=2
  Due Sample Start : Constant  Value=0
  Ready to Read : Constant  Value=0
  Uno Power : Constant  Value=0
  Outputs : Outport
  wires:
  RPM/1 -> Bus Creator/1  "RPM"
  Bus Creator/1 -> Bus Creator1/1  "Control Signals"
  Bus Creator2/1 -> Bus Creator/3  "Arduino Signals"
  Uno Power/1 -> Bus Creator2/2  "Uno Power"
  Desired Heading/1 -> Bus Creator/2  "Desired Heading"
  Bus Creator1/1 -> Bus Creator4/1  "Outputs"
  Annotated Image/1 -> Bus Creator1/2  "Annotated Image"
  Sensors/1 -> Bus Creator4/2  "Sensors"
  Bus Creator4/1 -> Bus Creator3/1  "Output Signals"
  Ready to Read/1 -> Bus Creator2/1  "Ready to Read"
  Due Sample Start/1 -> Bus Creator2/3  "Due Sample Start"
  Task Finished/1 -> Bus Creator3/2  "Task Finished"
  Bus Creator3/1 -> Outputs/1

== system RoboBoat_SLAM_6_29/Main FSM/Obstacle Navigation1/Enter Gate/Gate 2 (White & White)/Output Heirarchy ==
  Annotated Image : Inport
  Sensors : Inport  Port=2
  RPM : Inport  Port=3
  Desired Heading : Inport  Port=4
  Task Finished : Inport  Port=5
  Bus Creator : BusCreator  Inputs=3
  Bus Creator1 : BusCreator  Inputs=2
  Bus Creator2 : BusCreator  Inputs=3
  Bus Creator3 : BusCreator  Inputs=2
  Bus Creator4 : BusCreator  Inputs=2
  Due Sample Start : Constant  Value=0
  Ready to Read : Constant  Value=0
  Uno Power : Constant  Value=0
  Outputs : Outport
  wires:
  RPM/1 -> Bus Creator/1  "RPM"
  Bus Creator/1 -> Bus Creator1/1  "Control Signals"
  Bus Creator2/1 -> Bus Creator/3  "Arduino Signals"
  Uno Power/1 -> Bus Creator2/2  "Uno Power"
  Desired Heading/1 -> Bus Creator/2  "Desired Heading"
  Bus Creator1/1 -> Bus Creator4/1  "Outputs"
  Annotated Image/1 -> Bus Creator1/2  "Annotated Image"
  Sensors/1 -> Bus Creator4/2  "Sensors"
  Bus Creator4/1 -> Bus Creator3/1  "Output Signals"
  Ready to Read/1 -> Bus Creator2/1  "Ready to Read"
  Due Sample Start/1 -> Bus Creator2/3  "Due Sample Start"
  Task Finished/1 -> Bus Creator3/2  "Task Finished"
  Bus Creator3/1 -> Outputs/1

== system RoboBoat_SLAM_6_29/Main FSM/Obstacle Navigation1/Enter Gate/Gate 3 (White & Green)/Output Heirarchy ==
  Annotated Image : Inport
  Sensors : Inport  Port=2
  RPM : Inport  Port=3
  Desired Heading : Inport  Port=4
  Task Finished : Inport  Port=5
  Bus Creator : BusCreator  Inputs=3
  Bus Creator1 : BusCreator  Inputs=2
  Bus Creator2 : BusCreator  Inputs=3
  Bus Creator3 : BusCreator  Inputs=2
  Bus Creator4 : BusCreator  Inputs=2
  Due Sample Start : Constant  Value=0
  Ready to Read : Constant  Value=0
  Uno Power : Constant  Value=0
  Outputs : Outport
  wires:
  RPM/1 -> Bus Creator/1  "RPM"
  Bus Creator/1 -> Bus Creator1/1  "Control Signals"
  Bus Creator2/1 -> Bus Creator/3  "Arduino Signals"
  Uno Power/1 -> Bus Creator2/2  "Uno Power"
  Desired Heading/1 -> Bus Creator/2  "Desired Heading"
  Bus Creator1/1 -> Bus Creator4/1  "Outputs"
  Annotated Image/1 -> Bus Creator1/2  "Annotated Image"
  Sensors/1 -> Bus Creator4/2  "Sensors"
  Bus Creator4/1 -> Bus Creator3/1  "Output Signals"
  Ready to Read/1 -> Bus Creator2/1  "Ready to Read"
  Due Sample Start/1 -> Bus Creator2/3  "Due Sample Start"
  Task Finished/1 -> Bus Creator3/2  "Task Finished"
  Bus Creator3/1 -> Outputs/1

== system RoboBoat_SLAM_6_29/Main FSM/Obstacle Navigation1/Exit Gate/Gate 1 (Red & White)/Output Heirarchy ==
  Annotated Image : Inport
  Sensors : Inport  Port=2
  RPM : Inport  Port=3
  Desired Heading : Inport  Port=4
  Task Finished : Inport  Port=5
  Bus Creator : BusCreator  Inputs=3
  Bus Creator1 : BusCreator  Inputs=2
  Bus Creator2 : BusCreator  Inputs=3
  Bus Creator3 : BusCreator  Inputs=2
  Bus Creator4 : BusCreator  Inputs=2
  Due Sample Start : Constant  Value=0
  Ready to Read : Constant  Value=0
  Uno Power : Constant  Value=0
  Outputs : Outport
  wires:
  RPM/1 -> Bus Creator/1  "RPM"
  Bus Creator/1 -> Bus Creator1/1  "Control Signals"
  Bus Creator2/1 -> Bus Creator/3  "Arduino Signals"
  Uno Power/1 -> Bus Creator2/2  "Uno Power"
  Desired Heading/1 -> Bus Creator/2  "Desired Heading"
  Bus Creator1/1 -> Bus Creator4/1  "Outputs"
  Annotated Image/1 -> Bus Creator1/2  "Annotated Image"
  Sensors/1 -> Bus Creator4/2  "Sensors"
  Bus Creator4/1 -> Bus Creator3/1  "Output Signals"
  Ready to Read/1 -> Bus Creator2/1  "Ready to Read"
  Due Sample Start/1 -> Bus Creator2/3  "Due Sample Start"
  Task Finished/1 -> Bus Creator3/2  "Task Finished"
  Bus Creator3/1 -> Outputs/1

== system RoboBoat_SLAM_6_29/Main FSM/Obstacle Navigation1/Exit Gate/Gate 2 (White & White)/Output Heirarchy ==
  Annotated Image : Inport
  Sensors : Inport  Port=2
  RPM : Inport  Port=3
  Desired Heading : Inport  Port=4
  Task Finished : Inport  Port=5
  Bus Creator : BusCreator  Inputs=3
  Bus Creator1 : BusCreator  Inputs=2
  Bus Creator2 : BusCreator  Inputs=3
  Bus Creator3 : BusCreator  Inputs=2
  Bus Creator4 : BusCreator  Inputs=2
  Due Sample Start : Constant  Value=0
  Ready to Read : Constant  Value=0
  Uno Power : Constant  Value=0
  Outputs : Outport
  wires:
  RPM/1 -> Bus Creator/1  "RPM"
  Bus Creator/1 -> Bus Creator1/1  "Control Signals"
  Bus Creator2/1 -> Bus Creator/3  "Arduino Signals"
  Uno Power/1 -> Bus Creator2/2  "Uno Power"
  Desired Heading/1 -> Bus Creator/2  "Desired Heading"
  Bus Creator1/1 -> Bus Creator4/1  "Outputs"
  Annotated Image/1 -> Bus Creator1/2  "Annotated Image"
  Sensors/1 -> Bus Creator4/2  "Sensors"
  Bus Creator4/1 -> Bus Creator3/1  "Output Signals"
  Ready to Read/1 -> Bus Creator2/1  "Ready to Read"
  Due Sample Start/1 -> Bus Creator2/3  "Due Sample Start"
  Task Finished/1 -> Bus Creator3/2  "Task Finished"
  Bus Creator3/1 -> Outputs/1

== system RoboBoat_SLAM_6_29/Main FSM/Obstacle Navigation1/Exit Gate/Gate 3 (White & Green)/Output Heirarchy ==
  Annotated Image : Inport
  Sensors : Inport  Port=2
  RPM : Inport  Port=3
  Desired Heading : Inport  Port=4
  Task Finished : Inport  Port=5
  Bus Creator : BusCreator  Inputs=3
  Bus Creator1 : BusCreator  Inputs=2
  Bus Creator2 : BusCreator  Inputs=3
  Bus Creator3 : BusCreator  Inputs=2
  Bus Creator4 : BusCreator  Inputs=2
  Due Sample Start : Constant  Value=0
  Ready to Read : Constant  Value=0
  Uno Power : Constant  Value=0
  Outputs : Outport
  wires:
  RPM/1 -> Bus Creator/1  "RPM"
  Bus Creator/1 -> Bus Creator1/1  "Control Signals"
  Bus Creator2/1 -> Bus Creator/3  "Arduino Signals"
  Uno Power/1 -> Bus Creator2/2  "Uno Power"
  Desired Heading/1 -> Bus Creator/2  "Desired Heading"
  Bus Creator1/1 -> Bus Creator4/1  "Outputs"
  Annotated Image/1 -> Bus Creator1/2  "Annotated Image"
  Sensors/1 -> Bus Creator4/2  "Sensors"
  Bus Creator4/1 -> Bus Creator3/1  "Output Signals"
  Ready to Read/1 -> Bus Creator2/1  "Ready to Read"
  Due Sample Start/1 -> Bus Creator2/3  "Due Sample Start"
  Task Finished/1 -> Bus Creator3/2  "Task Finished"
  Bus Creator3/1 -> Outputs/1

== system RoboBoat_SLAM_6_29/Main FSM/Obstacle Navigation1/GPS: Center/Approach/Output Heirarchy ==
  Finished : Inport
  Desired Heading : Inport  Port=2
  Annotated Image : Inport  Port=3
  Sensors : Inport  Port=4
  Bus Creator : BusCreator  Inputs=3
  Bus Creator1 : BusCreator  Inputs=2
  Bus Creator2 : BusCreator  Inputs=3
  Bus Creator3 : BusCreator  Inputs=2
  Bus Creator4 : BusCreator  Inputs=2
  Due Sample Start : Constant  Value=0
  RPM Desired : Constant  Value=4000
  Ready to Read : Constant  Value=0
  Uno Power : Constant  Value=0
  Outputs : Outport
  wires:
  RPM Desired/1 -> Bus Creator/1  "RPM"
  Bus Creator/1 -> Bus Creator1/1  "Control Signals"
  Bus Creator2/1 -> Bus Creator/3  "Arduino Signals"
  Uno Power/1 -> Bus Creator2/2  "Uno Power"
  Desired Heading/1 -> Bus Creator/2  "Desired Heading"
  Bus Creator1/1 -> Bus Creator4/1  "Outputs"
  Annotated Image/1 -> Bus Creator1/2  "Annotated Image"
  Sensors/1 -> Bus Creator4/2  "Sensors"
  Bus Creator4/1 -> Bus Creator3/1  "Output Signals"
  Ready to Read/1 -> Bus Creator2/1  "Ready to Read"
  Due Sample Start/1 -> Bus Creator2/3  "Due Sample Start"
  Bus Creator3/1 -> Outputs/1
  Finished/1 -> Bus Creator3/2  "Task Finished"

== system RoboBoat_SLAM_6_29/Main FSM/Obstacle Navigation1/GPS: Center/Orient/Output Heirarchy1 ==
  Annotated Image : Inport
  Desired Heading : Inport  Port=2
  Sensors : Inport  Port=3
  Bus Creator : BusCreator  Inputs=3
  Bus Creator1 : BusCreator  Inputs=2
  Bus Creator2 : BusCreator  Inputs=3
  Bus Creator3 : BusCreator  Inputs=2
  Bus Creator4 : BusCreator  Inputs=2
  Due Sample Start : Constant  Value=0
  Finished : Constant  Value=0
  RPM Desired : Constant  Value=0
  Ready to Read : Constant  Value=0
  Uno Power : Constant  Value=0
  Outputs : Outport
  wires:
  RPM Desired/1 -> Bus Creator/1  "RPM"
  Bus Creator/1 -> Bus Creator1/1  "Control Signals"
  Bus Creator2/1 -> Bus Creator/3  "Arduino Signals"
  Uno Power/1 -> Bus Creator2/2  "Uno Power"
  Desired Heading/1 -> Bus Creator/2  "Desired Heading"
  Bus Creator1/1 -> Bus Creator4/1  "Outputs"
  Annotated Image/1 -> Bus Creator1/2  "Annotated Image"
  Sensors/1 -> Bus Creator4/2  "Sensors"
  Bus Creator4/1 -> Bus Creator3/1  "Output Signals"
  Ready to Read/1 -> Bus Creator2/1  "Ready to Read"
  Due Sample Start/1 -> Bus Creator2/3  "Due Sample Start"
  Bus Creator3/1 -> Outputs/1
  Finished/1 -> Bus Creator3/2  "Task Finished"

== system RoboBoat_SLAM_6_29/Main FSM/Obstacle Navigation1/Obstacle Navigation/Dodge/Output Heirarchy ==
  Annotated Image : Inport
  Sensors : Inport  Port=2
  RPM : Inport  Port=3
  Desired Heading : Inport  Port=4
  Bus Creator : BusCreator  Inputs=3
  Bus Creator1 : BusCreator  Inputs=2
  Bus Creator2 : BusCreator  Inputs=3
  Bus Creator3 : BusCreator  Inputs=2
  Bus Creator4 : BusCreator  Inputs=2
  Due Sample Start : Constant  Value=0
  Nav Finished : Constant  Value=0
  Ready to Read : Constant  Value=0
  Uno Power : Constant  Value=0
  Outputs : Outport
  wires:
  RPM/1 -> Bus Creator/1  "RPM"
  Bus Creator/1 -> Bus Creator1/1  "Control Signals"
  Bus Creator2/1 -> Bus Creator/3  "Arduino Signals"
  Uno Power/1 -> Bus Creator2/2  "Uno Power"
  Desired Heading/1 -> Bus Creator/2  "Desired Heading"
  Bus Creator1/1 -> Bus Creator4/1  "Outputs"
  Annotated Image/1 -> Bus Creator1/2  "Annotated Image"
  Sensors/1 -> Bus Creator4/2  "Sensors"
  Bus Creator4/1 -> Bus Creator3/1  "Output Signals"
  Ready to Read/1 -> Bus Creator2/1  "Ready to Read"
  Due Sample Start/1 -> Bus Creator2/3  "Due Sample Start"
  Bus Creator3/1 -> Outputs/1
  Nav Finished/1 -> Bus Creator3/2  "Task Finished"

== system RoboBoat_SLAM_6_29/Main FSM/Obstacle Navigation1/Obstacle Navigation/GPS: Bee Line/Approach ==
  Sensors : Inport
  RGB image : Inport  Port=2
  Enable : EnablePort
  Annotate Task : visiontextngfix/Insert Text  inputType=Obsolete  theText='GPS - Start: Approach - Distance: %f'  getTextLocFrom=Specify via dialog  textLoc=[10 70]  getTextColorFrom=Specify via dialog  textColor=[255 0 0]  getTextIntensityFrom=Specify via dialog  textIntensity=0  getTextOpacityFrom=Specify via dialog  textOpacity=1.0  dummyVar2=0  dummyVar3=0  dummyVar4=0  imagePorts=One multidimensional signal  isInputTransposed=off  fontFace=LucidaSansRegular  dummyVar1=0  blockFontSize=12  antiAliased=on
  Annotate Task2 : visiontextngfix/Insert Text  inputType=Obsolete  theText='Bee Line Approach'  getTextLocFrom=Specify via dialog  textLoc=[1 1]  getTextColorFrom=Specify via dialog  textColor=[0 0 0]  getTextIntensityFrom=Specify via dialog  textIntensity=0  getTextOpacityFrom=Specify via dialog  textOpacity=1.0  dummyVar2=0  dummyVar3=0  dummyVar4=0  imagePorts=One multidimensional signal  isInputTransposed=off  fontFace=LucidaSansRegular  dummyVar1=0  blockFontSize=12  antiAliased=on
  Annotate Task3 : visiontextngfix/Insert Text  inputType=Obsolete  theText='Obstacle- Distance: %f'  getTextLocFrom=Specify via dialog  textLoc=[10 100]  getTextColorFrom=Specify via dialog  textColor=[255 0 0]  getTextIntensityFrom=Specify via dialog  textIntensity=0  getTextOpacityFrom=Specify via dialog  textOpacity=1.0  dummyVar2=0  dummyVar3=0  dummyVar4=0  imagePorts=One multidimensional signal  isInputTransposed=off  fontFace=LucidaSansRegular  dummyVar1=0  blockFontSize=12  antiAliased=on
  Bus Selector : BusSelector  OutputSignals=Serial In.GPS.latitude,Serial In.GPS.longitude,Serial In.Buoy Info.Color ID,Serial In.Buoy Info.Distance
  Compare To Constant : simulink/Logic and Bit Operations/Compare To Constant  relop=<=  const=5  OutDataTypeStr=boolean
  Data Store Read : DataStoreRead  DataStoreName=obstNavEndGPS  SampleTime=0.1
  Data Type Conversion : DataTypeConversion  OutDataTypeStr=double
  Desired Heading and Distance : MATLAB Function  TreatAsAtomicUnit=on
  Obstacle Distance : MATLAB Function  TreatAsAtomicUnit=on
  Output Heirarchy : Subsystem
  Outputs : Outport
  Dodge Start : Outport  Port=2
  wires:
  Sensors/1 -> Output Heirarchy/3(Sensors), Bus Selector/1  "Sensors"
  Data Store Read/1 -> Desired Heading and Distance/1(DesiredGPS)
  Bus Selector/1 -> Desired Heading and Distance/2(GPSLat)  "<latitude>"
  Bus Selector/2 -> Desired Heading and Distance/3(GPSLong)  "<longitude>"
  Desired Heading and Distance/2(DesiredHeading) -> Output Heirarchy/2(Desired Heading)
  RGB image/1 -> Annotate Task2/1
  Desired Heading and Distance/1(Distance) -> Compare To Constant/1, Annotate Task/2
  Data Type Conversion/1 -> Output Heirarchy/1(Nav Finished)  "Task Finished"
  Output Heirarchy/1(Outputs) -> Outputs/1
  Annotate Task2/1 -> Annotate Task/1
  Annotate Task/1 -> Annotate Task3/1
  Annotate Task3/1 -> Output Heirarchy/4(Annotated Image)
  Obstacle Distance/2(DodgeStart) -> Dodge Start/1
  Compare To Constant/1 -> Data Type Conversion/1
  Obstacle Distance/1(ObstDist) -> Annotate Task3/2
  Bus Selector/3 -> Obstacle Distance/1(ColorID)  "<Color ID>"
  Bus Selector/4 -> Obstacle Distance/2(Dist)  "<Distance>"

== system RoboBoat_SLAM_6_29/Main FSM/Obstacle Navigation1/Obstacle Navigation/GPS: Bee Line/Orient ==
  Sensors : Inport
  RGB image : Inport  Port=2
  Enable : EnablePort
  Annotate Task : visiontextngfix/Insert Text  inputType=Obsolete  theText='GPS - Center: Orient %f'  getTextLocFrom=Specify via dialog  textLoc=[10 70]  getTextColorFrom=Specify via dialog  textColor=[255 0 0]  getTextIntensityFrom=Specify via dialog  textIntensity=0  getTextOpacityFrom=Specify via dialog  textOpacity=1.0  dummyVar2=0  dummyVar3=0  dummyVar4=0  imagePorts=One multidimensional signal  isInputTransposed=off  fontFace=LucidaSansRegular  dummyVar1=0  blockFontSize=12  antiAliased=on
  Annotate Task1 : visiontextngfix/Insert Text  inputType=Obsolete  theText='Current Heading %f'  getTextLocFrom=Specify via dialog  textLoc=[10 40]  getTextColorFrom=Specify via dialog  textColor=[255 0 0]  getTextIntensityFrom=Specify via dialog  textIntensity=0  getTextOpacityFrom=Specify via dialog  textOpacity=1.0  dummyVar2=0  dummyVar3=0  dummyVar4=0  imagePorts=One multidimensional signal  isInputTransposed=off  fontFace=LucidaSansRegular  dummyVar1=0  blockFontSize=12  antiAliased=on
  Annotate Task2 : visiontextngfix/Insert Text  inputType=Obsolete  theText='Bee Line Orient'  getTextLocFrom=Specify via dialog  textLoc=[1 1]  getTextColorFrom=Specify via dialog  textColor=[0 0 0]  getTextIntensityFrom=Specify via dialog  textIntensity=0  getTextOpacityFrom=Specify via dialog  textOpacity=1.0  dummyVar2=0  dummyVar3=0  dummyVar4=0  imagePorts=One multidimensional signal  isInputTransposed=off  fontFace=LucidaSansRegular  dummyVar1=0  blockFontSize=12  antiAliased=on
  Bus Selector : BusSelector  OutputSignals=Serial In.GPS.latitude,Serial In.GPS.longitude,Serial In.Compass.Heading
  Data Store Read1 : DataStoreRead  DataStoreName=obstNavEndGPS  SampleTime=0.1
  Desired Heading : MATLAB Function  TreatAsAtomicUnit=on
  Output Heirarchy1 : Subsystem
  Within Range : MATLAB Function  TreatAsAtomicUnit=on
  Outputs : Outport
  Finished : Outport  Port=2
  wires:
  Sensors/1 -> Output Heirarchy1/3(Sensors), Bus Selector/1  "Sensors"
  Data Store Read1/1 -> Desired Heading/1(DesiredGPS)
  Bus Selector/1 -> Desired Heading/2(GPSLat)  "<latitude>"
  Bus Selector/2 -> Desired Heading/3(GPSLong)  "<longitude>"
  Desired Heading/1(DesiredHeading) -> Output Heirarchy1/2(Desired Heading), Annotate Task/2, Within Range/1(DesiredHeading)
  Bus Selector/3 -> Annotate Task1/2, Within Range/2(Compass)  "<Heading>"
  Within Range/1(Finished) -> Finished/1
  RGB image/1 -> Annotate Task2/1
  Output Heirarchy1/1(Outputs) -> Outputs/1
  Annotate Task/1 -> Annotate Task1/1
  Annotate Task1/1 -> Output Heirarchy1/1(Annotated Image)
  Annotate Task2/1 -> Annotate Task/1
